simulink model "AuM_Ha5_A1"  (R2020a)
settings: Solver=VariableStepAuto  StartTime=0.0  StopTime=5  RelTol=1e-9
values from neighbouring files (symbols this model uses):
  J = 450e-6    (= 0.00045)    [AuM_HA05_A1_init.m]    (also in AuM_HA05_A2_init.m)
  L_S = 4e-3    (= 0.004)    [AuM_HA05_A1_init.m]    (also in AuM_HA05_A2_init.m)
  p = 5    [AuM_HA05_A1_init.m]    (also in AuM_HA05_A2_init.m)
  Psi_P = 4.5e-3    (= 0.0045)    [AuM_HA05_A1_init.m]    (also in AuM_HA05_A2_init.m)
  R_S = 0.58    [AuM_HA05_A1_init.m]    (also in AuM_HA05_A2_init.m)
  T_S = L_S/R_S    (= 0.00689655172414)    [AuM_HA05_A1_init.m]    (also in AuM_HA05_A2_init.m)
  U_d = 24    [AuM_HA05_A1_init.m]    (also in AuM_HA05_A2_init.m)
settings Model: Creator=Ravi Plenzdorf  LastModifiedBy=Ravi Plenzdorf

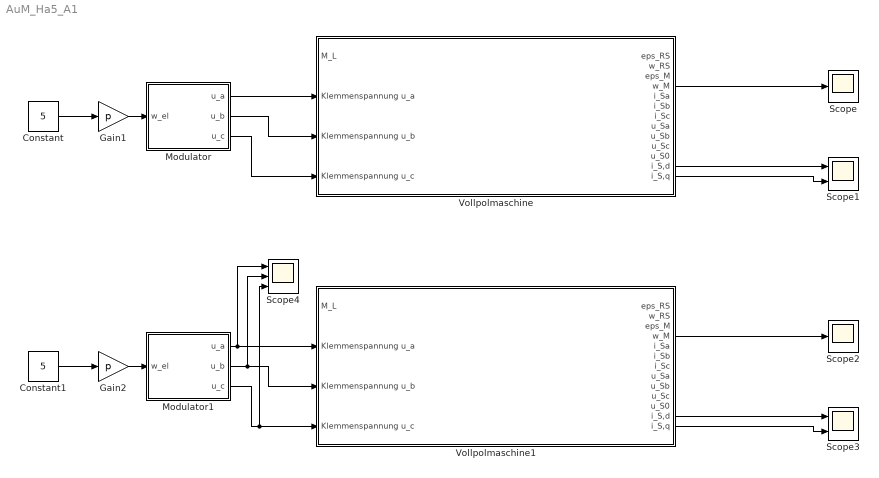
== system AuM_Ha5_A1 ==
  Constant : Constant  Value=5
  Constant1 : Constant  Value=5
  Gain1 : Gain  Gain=p
  Gain2 : Gain  Gain=p
  Modulator : Subsystem
  Modulator1 : Subsystem
  Scope : Scope
  Scope1 : Scope  NumInputPorts=2
  Scope2 : Scope
  Scope3 : Scope  NumInputPorts=2
  Scope4 : Scope  NumInputPorts=3
  Vollpolmaschine : Subsystem
      mask Display: image('Motor_Symbol.png'); % Use "Edit Image" on toolstrip to change.
  Vollpolmaschine1 : Subsystem
      mask Display: image('Motor_Symbol.png'); % Use "Edit Image" on toolstrip to change.
  wires:
  Vollpolmaschine/4(w_M) -> Scope/1
  Vollpolmaschine/12(i_S,d) -> Scope1/1
  Vollpolmaschine/13(i_S,q) -> Scope1/2
  Constant/1 -> Gain1/1
  Gain1/1 -> Modulator/1(w_el)
  Modulator/1(u_a) -> Vollpolmaschine/2(Klemmenspannung u_a)
  Modulator/2(u_b) -> Vollpolmaschine/3(Klemmenspannung u_b)
  Modulator/3(u_c) -> Vollpolmaschine/4(Klemmenspannung u_c)
  Modulator1/3(u_c) -> Scope4/3, Vollpolmaschine1/4(Klemmenspannung u_c)
  Modulator1/2(u_b) -> Scope4/2, Vollpolmaschine1/3(Klemmenspannung u_b)
  Modulator1/1(u_a) -> Vollpolmaschine1/2(Klemmenspannung u_a), Scope4/1
  Gain2/1 -> Modulator1/1(w_el)
  Constant1/1 -> Gain2/1
  Vollpolmaschine1/13(i_S,q) -> Scope3/2
  Vollpolmaschine1/12(i_S,d) -> Scope3/1
  Vollpolmaschine1/4(w_M) -> Scope2/1

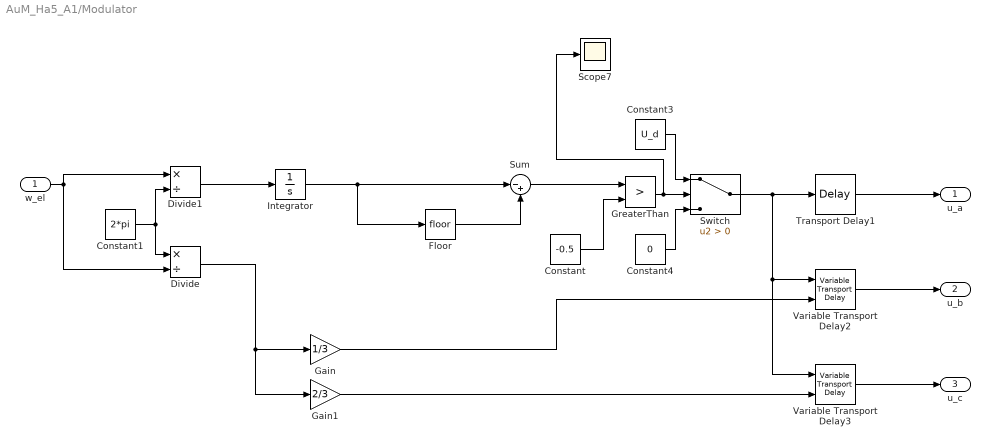
== system AuM_Ha5_A1/Modulator ==
  w_el : Inport
  Constant : Constant  Value=-0.5
  Constant1 : Constant  Value=2*pi
  Constant3 : Constant  Value=U_d
  Constant4 : Constant  Value=0
  Divide : Product  Inputs=*/
  Divide1 : Product  Inputs=*/
  Floor : Rounding
  Gain : Gain  Gain=1/3
  Gain1 : Gain  Gain=2/3
  GreaterThan : RelationalOperator  Operator=>  OutDataTypeStr=boolean  RndMeth=Simplest
  Integrator : Integrator
  Scope7 : Scope
  Sum : Sum  Inputs=|-+
  Switch : Switch  Criteria=u2 > Threshold
  Transport Delay1 : TransportDelay  DelayTime=0
  Variable Transport Delay2 : VariableTransportDelay  VariableDelayType=Variable transport delay  MaximumDelay=10
  Variable Transport Delay3 : VariableTransportDelay  VariableDelayType=Variable transport delay  MaximumDelay=10
  u_a : Outport
  u_b : Outport  Port=2
  u_c : Outport  Port=3
  wires:
  Constant4/1 -> Switch/3
  Constant3/1 -> Switch/1
  Sum/1 -> GreaterThan/1
  GreaterThan/1 -> Scope7/1, Switch/2
  Constant/1 -> GreaterThan/2
  Integrator/1 -> Floor/1, Sum/1
  Floor/1 -> Sum/2
  Switch/1 -> Variable Transport Delay3/1, Variable Transport Delay2/1, Transport Delay1/1
  w_el/1 -> Divide1/1, Divide/2
  Divide/1 -> Gain1/1, Gain/1
  Gain/1 -> Variable Transport Delay2/2
  Gain1/1 -> Variable Transport Delay3/2
  Constant1/1 -> Divide/1, Divide1/2
  Divide1/1 -> Integrator/1
  Transport Delay1/1 -> u_a/1
  Variable Transport Delay2/1 -> u_b/1
  Variable Transport Delay3/1 -> u_c/1

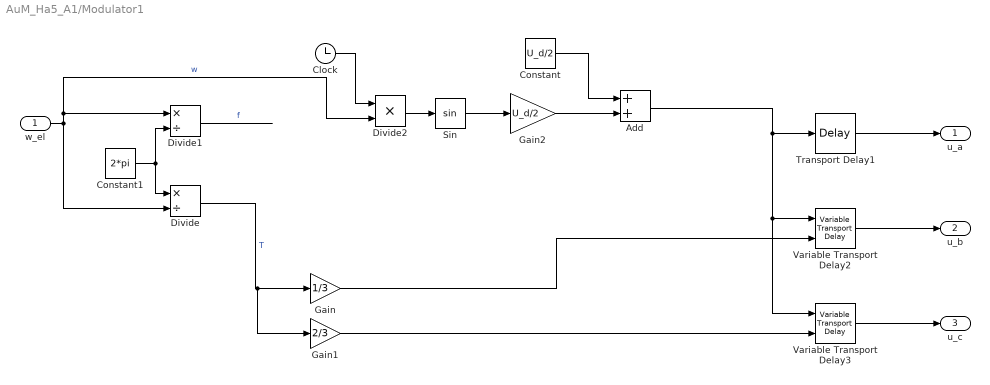
== system AuM_Ha5_A1/Modulator1 ==
  w_el : Inport
  Add : Sum
  Clock : Clock
  Constant : Constant  Value=U_d/2
  Constant1 : Constant  Value=2*pi
  Divide : Product  Inputs=*/
  Divide1 : Product  Inputs=*/
  Divide2 : Product  Inputs=**
  Gain : Gain  Gain=1/3
  Gain1 : Gain  Gain=2/3
  Gain2 : Gain  Gain=U_d/2
  Sin : Trigonometry
  Transport Delay1 : TransportDelay  DelayTime=0
  Variable Transport Delay2 : VariableTransportDelay  VariableDelayType=Variable transport delay  MaximumDelay=10
  Variable Transport Delay3 : VariableTransportDelay  VariableDelayType=Variable transport delay  MaximumDelay=10
  u_a : Outport
  u_b : Outport  Port=2
  u_c : Outport  Port=3
  wires:
  Variable Transport Delay3/1 -> u_c/1
  Variable Transport Delay2/1 -> u_b/1
  Transport Delay1/1 -> u_a/1
  Constant1/1 -> Divide1/2, Divide/1
  Gain/1 -> Variable Transport Delay2/2
  w_el/1 -> Divide2/2, Divide1/1, Divide/2  "w"
  Add/1 -> Transport Delay1/1, Variable Transport Delay2/1, Variable Transport Delay3/1
  Divide/1 -> Gain1/1, Gain/1  "T"
  Divide1/1 -> ?  "f"
  Gain1/1 -> Variable Transport Delay3/2
  Clock/1 -> Divide2/1
  Divide2/1 -> Sin/1
  Sin/1 -> Gain2/1
  Gain2/1 -> Add/2
  Constant/1 -> Add/1

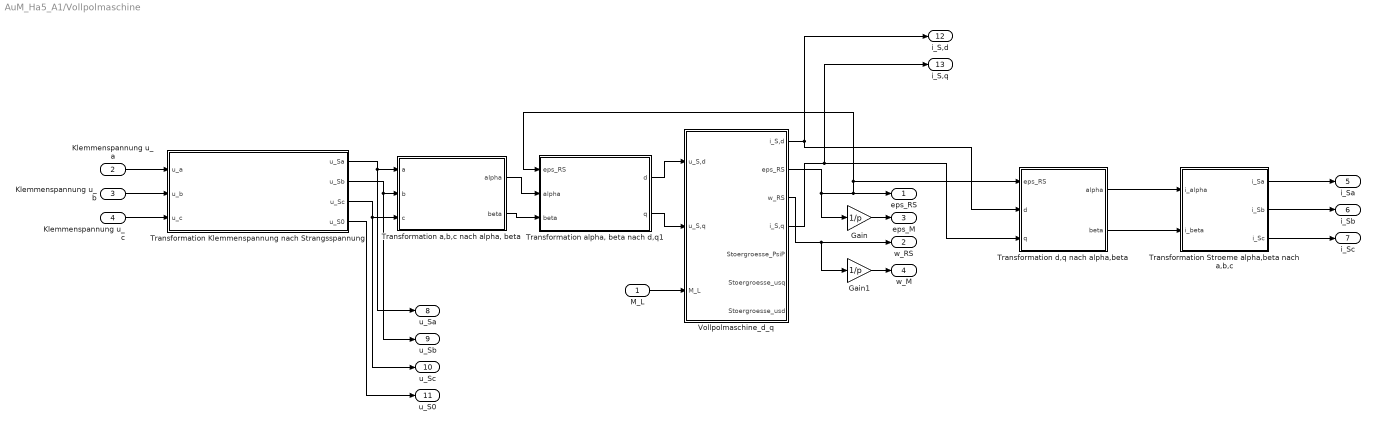
== system AuM_Ha5_A1/Vollpolmaschine ==
  M_L : Inport
  Klemmenspannung u_a : Inport  Port=2
  Klemmenspannung u_b : Inport  Port=3
  Klemmenspannung u_c : Inport  Port=4
  Gain : Gain  Gain=1/p
  Gain1 : Gain  Gain=1/p
  Transformation Klemmenspannung nach Strangsspannung : MATLAB Function  TreatAsAtomicUnit=on
  Transformation Stroeme alpha,beta nach a,b,c : MATLAB Function  TreatAsAtomicUnit=on
  "Transformation a,b,c nach alpha, beta" : MATLAB Function  TreatAsAtomicUnit=on
  "Transformation alpha, beta nach d,q1" : MATLAB Function  TreatAsAtomicUnit=on
  Transformation d,q nach alpha,beta : MATLAB Function  TreatAsAtomicUnit=on
  Vollpolmaschine_d_q : Subsystem
  eps_RS : Outport  VectorParamsAs1DForOutWhenUnconnected=off
  w_RS : Outport  Port=2  VectorParamsAs1DForOutWhenUnconnected=off
  eps_M : Outport  Port=3  VectorParamsAs1DForOutWhenUnconnected=off
  w_M : Outport  Port=4  VectorParamsAs1DForOutWhenUnconnected=off
  i_Sa : Outport  Port=5  VectorParamsAs1DForOutWhenUnconnected=off
  i_Sb : Outport  Port=6  VectorParamsAs1DForOutWhenUnconnected=off
  i_Sc : Outport  Port=7  VectorParamsAs1DForOutWhenUnconnected=off
  u_Sa : Outport  Port=8  VectorParamsAs1DForOutWhenUnconnected=off
  u_Sb : Outport  Port=9  VectorParamsAs1DForOutWhenUnconnected=off
  u_Sc : Outport  Port=10  VectorParamsAs1DForOutWhenUnconnected=off
  u_S0 : Outport  Port=11  VectorParamsAs1DForOutWhenUnconnected=off
  i_S,d : Outport  Port=12
  i_S,q : Outport  Port=13
  wires:
  Transformation Klemmenspannung nach Strangsspannung/4(u_S0) -> u_S0/1
  Transformation Stroeme alpha,beta nach a,b,c/3(i_Sc) -> i_Sc/1
  Transformation Stroeme alpha,beta nach a,b,c/2(i_Sb) -> i_Sb/1
  Transformation Stroeme alpha,beta nach a,b,c/1(i_Sa) -> i_Sa/1
  Transformation d,q nach alpha,beta/2(beta) -> Transformation Stroeme alpha,beta nach a,b,c/2(i_beta)
  Transformation d,q nach alpha,beta/1(alpha) -> Transformation Stroeme alpha,beta nach a,b,c/1(i_alpha)
  "Transformation alpha, beta nach d,q1"/1(d) -> Vollpolmaschine_d_q/1(u_S,d)
  Gain1/1 -> w_M/1
  Gain/1 -> eps_M/1
  Klemmenspannung u_c/1 -> Transformation Klemmenspannung nach Strangsspannung/3(u_c)
  Klemmenspannung u_b/1 -> Transformation Klemmenspannung nach Strangsspannung/2(u_b)
  Klemmenspannung u_a/1 -> Transformation Klemmenspannung nach Strangsspannung/1(u_a)
  "Transformation alpha, beta nach d,q1"/2(q) -> Vollpolmaschine_d_q/2(u_S,q)
  "Transformation a,b,c nach alpha, beta"/2(beta) -> "Transformation alpha, beta nach d,q1"/3(beta)
  "Transformation a,b,c nach alpha, beta"/1(alpha) -> "Transformation alpha, beta nach d,q1"/2(alpha)
  M_L/1 -> Vollpolmaschine_d_q/3(M_L)
  Transformation Klemmenspannung nach Strangsspannung/3(u_Sc) -> u_Sc/1, "Transformation a,b,c nach alpha, beta"/3(c)
  Vollpolmaschine_d_q/2(eps_RS) -> Gain/1, "Transformation alpha, beta nach d,q1"/1(eps_RS), Transformation d,q nach alpha,beta/1(eps_RS), eps_RS/1
  Transformation Klemmenspannung nach Strangsspannung/1(u_Sa) -> "Transformation a,b,c nach alpha, beta"/1(a), u_Sa/1
  Vollpolmaschine_d_q/3(w_RS) -> w_RS/1, Gain1/1
  Transformation Klemmenspannung nach Strangsspannung/2(u_Sb) -> "Transformation a,b,c nach alpha, beta"/2(b), u_Sb/1
  Vollpolmaschine_d_q/1(i_S,d) -> Transformation d,q nach alpha,beta/2(d), i_S,d/1
  Vollpolmaschine_d_q/4(i_S,q) -> Transformation d,q nach alpha,beta/3(q), i_S,q/1

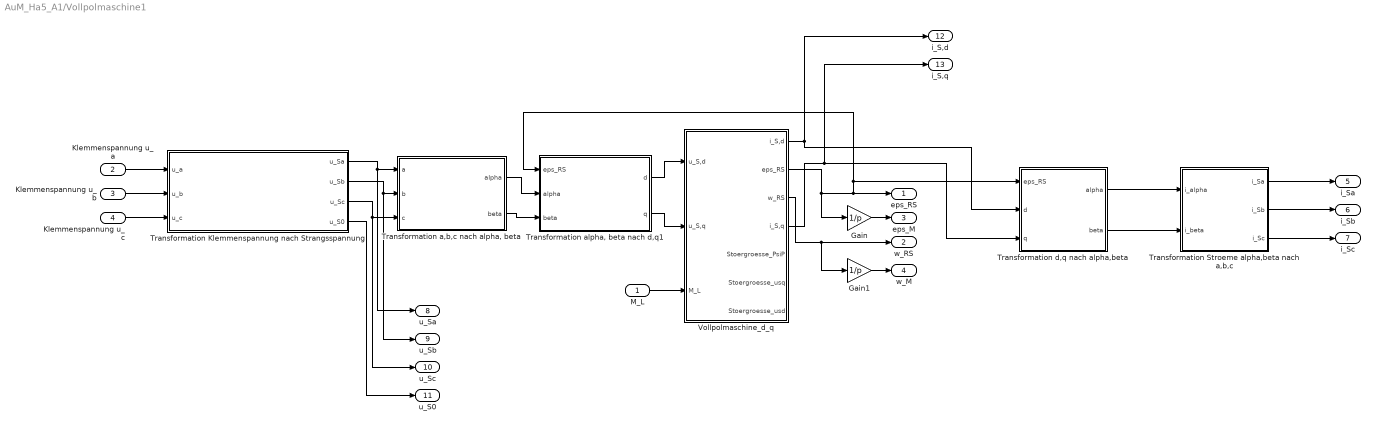
== system AuM_Ha5_A1/Vollpolmaschine1 ==
  M_L : Inport
  Klemmenspannung u_a : Inport  Port=2
  Klemmenspannung u_b : Inport  Port=3
  Klemmenspannung u_c : Inport  Port=4
  Gain : Gain  Gain=1/p
  Gain1 : Gain  Gain=1/p
  Transformation Klemmenspannung nach Strangsspannung : MATLAB Function  TreatAsAtomicUnit=on
  Transformation Stroeme alpha,beta nach a,b,c : MATLAB Function  TreatAsAtomicUnit=on
  "Transformation a,b,c nach alpha, beta" : MATLAB Function  TreatAsAtomicUnit=on
  "Transformation alpha, beta nach d,q1" : MATLAB Function  TreatAsAtomicUnit=on
  Transformation d,q nach alpha,beta : MATLAB Function  TreatAsAtomicUnit=on
  Vollpolmaschine_d_q : Subsystem
  eps_RS : Outport  VectorParamsAs1DForOutWhenUnconnected=off
  w_RS : Outport  Port=2  VectorParamsAs1DForOutWhenUnconnected=off
  eps_M : Outport  Port=3  VectorParamsAs1DForOutWhenUnconnected=off
  w_M : Outport  Port=4  VectorParamsAs1DForOutWhenUnconnected=off
  i_Sa : Outport  Port=5  VectorParamsAs1DForOutWhenUnconnected=off
  i_Sb : Outport  Port=6  VectorParamsAs1DForOutWhenUnconnected=off
  i_Sc : Outport  Port=7  VectorParamsAs1DForOutWhenUnconnected=off
  u_Sa : Outport  Port=8  VectorParamsAs1DForOutWhenUnconnected=off
  u_Sb : Outport  Port=9  VectorParamsAs1DForOutWhenUnconnected=off
  u_Sc : Outport  Port=10  VectorParamsAs1DForOutWhenUnconnected=off
  u_S0 : Outport  Port=11  VectorParamsAs1DForOutWhenUnconnected=off
  i_S,d : Outport  Port=12
  i_S,q : Outport  Port=13
  wires:
  Vollpolmaschine_d_q/4(i_S,q) -> i_S,q/1, Transformation d,q nach alpha,beta/3(q)
  Vollpolmaschine_d_q/1(i_S,d) -> i_S,d/1, Transformation d,q nach alpha,beta/2(d)
  Transformation Klemmenspannung nach Strangsspannung/2(u_Sb) -> u_Sb/1, "Transformation a,b,c nach alpha, beta"/2(b)
  Vollpolmaschine_d_q/3(w_RS) -> Gain1/1, w_RS/1
  Transformation Klemmenspannung nach Strangsspannung/1(u_Sa) -> u_Sa/1, "Transformation a,b,c nach alpha, beta"/1(a)
  Vollpolmaschine_d_q/2(eps_RS) -> eps_RS/1, Transformation d,q nach alpha,beta/1(eps_RS), "Transformation alpha, beta nach d,q1"/1(eps_RS), Gain/1
  Transformation Klemmenspannung nach Strangsspannung/3(u_Sc) -> "Transformation a,b,c nach alpha, beta"/3(c), u_Sc/1
  M_L/1 -> Vollpolmaschine_d_q/3(M_L)
  "Transformation a,b,c nach alpha, beta"/1(alpha) -> "Transformation alpha, beta nach d,q1"/2(alpha)
  "Transformation a,b,c nach alpha, beta"/2(beta) -> "Transformation alpha, beta nach d,q1"/3(beta)
  "Transformation alpha, beta nach d,q1"/2(q) -> Vollpolmaschine_d_q/2(u_S,q)
  Klemmenspannung u_a/1 -> Transformation Klemmenspannung nach Strangsspannung/1(u_a)
  Klemmenspannung u_b/1 -> Transformation Klemmenspannung nach Strangsspannung/2(u_b)
  Klemmenspannung u_c/1 -> Transformation Klemmenspannung nach Strangsspannung/3(u_c)
  Gain/1 -> eps_M/1
  Gain1/1 -> w_M/1
  "Transformation alpha, beta nach d,q1"/1(d) -> Vollpolmaschine_d_q/1(u_S,d)
  Transformation d,q nach alpha,beta/1(alpha) -> Transformation Stroeme alpha,beta nach a,b,c/1(i_alpha)
  Transformation d,q nach alpha,beta/2(beta) -> Transformation Stroeme alpha,beta nach a,b,c/2(i_beta)
  Transformation Stroeme alpha,beta nach a,b,c/1(i_Sa) -> i_Sa/1
  Transformation Stroeme alpha,beta nach a,b,c/2(i_Sb) -> i_Sb/1
  Transformation Stroeme alpha,beta nach a,b,c/3(i_Sc) -> i_Sc/1
  Transformation Klemmenspannung nach Strangsspannung/4(u_S0) -> u_S0/1

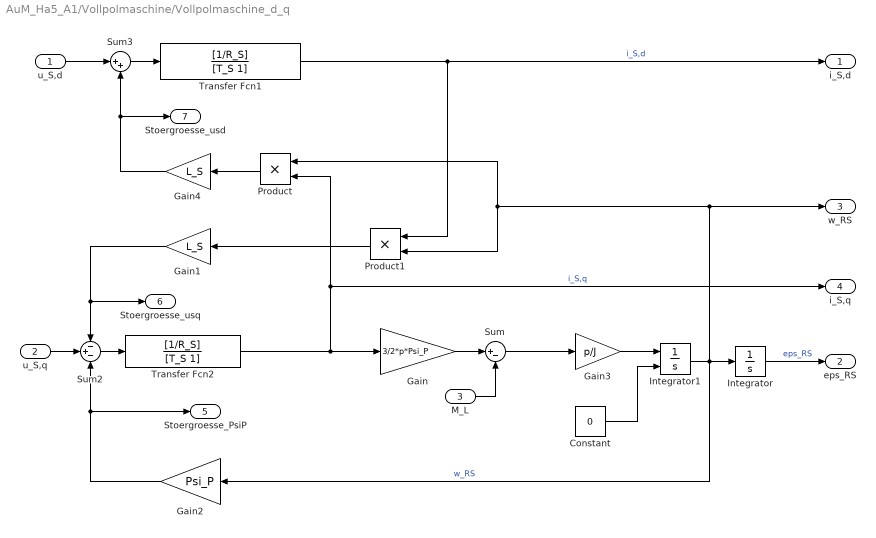
== system AuM_Ha5_A1/Vollpolmaschine/Vollpolmaschine_d_q ==
  u_S,d : Inport
  u_S,q : Inport  Port=2
  M_L : Inport  Port=3
  Constant : Constant  Value=0
  Gain : Gain  Gain=3/2*p*Psi_P
  Gain1 : Gain  Gain=L_S
  Gain2 : Gain  Gain=Psi_P
  Gain3 : Gain  Gain=p/J
  Gain4 : Gain  Gain=L_S
  Integrator : Integrator
  Integrator1 : Integrator  InitialConditionSource=external
  Product : Product
  Product1 : Product
  Sum : Sum  Inputs=|+-
  Sum2 : Sum  Inputs=-+-
  Sum3 : Sum  Inputs=|++
  Transfer Fcn1 : TransferFcn  Numerator=[1/R_S]  Denominator=[T_S 1]
  Transfer Fcn2 : TransferFcn  Numerator=[1/R_S]  Denominator=[T_S 1]
  i_S,d : Outport  VectorParamsAs1DForOutWhenUnconnected=off
  eps_RS : Outport  Port=2  VectorParamsAs1DForOutWhenUnconnected=off
  w_RS : Outport  Port=3  VectorParamsAs1DForOutWhenUnconnected=off
  i_S,q : Outport  Port=4  VectorParamsAs1DForOutWhenUnconnected=off
  Stoergroesse_PsiP : Outport  Port=5  VectorParamsAs1DForOutWhenUnconnected=off
  Stoergroesse_usq : Outport  Port=6  VectorParamsAs1DForOutWhenUnconnected=off
  Stoergroesse_usd : Outport  Port=7  VectorParamsAs1DForOutWhenUnconnected=off
  wires:
  Constant/1 -> Integrator1/2
  Transfer Fcn2/1 -> Product/2, i_S,q/1, Gain/1  "i_S,q"
  Gain4/1 -> Sum3/2, Stoergroesse_usd/1
  u_S,d/1 -> Sum3/1
  Gain1/1 -> Sum2/1, Stoergroesse_usq/1
  u_S,q/1 -> Sum2/2
  Product1/1 -> Gain1/1
  Transfer Fcn1/1 -> Product1/1, i_S,d/1  "i_S,d"
  Product/1 -> Gain4/1
  Sum3/1 -> Transfer Fcn1/1
  Gain2/1 -> Sum2/3, Stoergroesse_PsiP/1
  Gain3/1 -> Integrator1/1
  Gain/1 -> Sum/1
  M_L/1 -> Sum/2
  Sum/1 -> Gain3/1
  Integrator/1 -> eps_RS/1  "eps_RS"
  Integrator1/1 -> Gain2/1, Product1/2, Product/1, w_RS/1, Integrator/1  "w_RS"
  Sum2/1 -> Transfer Fcn2/1

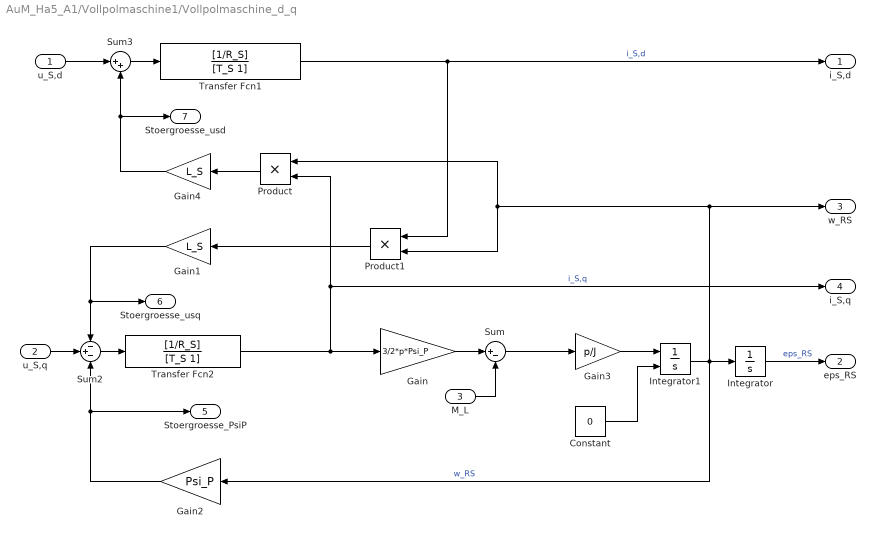
== system AuM_Ha5_A1/Vollpolmaschine1/Vollpolmaschine_d_q ==
  u_S,d : Inport
  u_S,q : Inport  Port=2
  M_L : Inport  Port=3
  Constant : Constant  Value=0
  Gain : Gain  Gain=3/2*p*Psi_P
  Gain1 : Gain  Gain=L_S
  Gain2 : Gain  Gain=Psi_P
  Gain3 : Gain  Gain=p/J
  Gain4 : Gain  Gain=L_S
  Integrator : Integrator
  Integrator1 : Integrator  InitialConditionSource=external
  Product : Product
  Product1 : Product
  Sum : Sum  Inputs=|+-
  Sum2 : Sum  Inputs=-+-
  Sum3 : Sum  Inputs=|++
  Transfer Fcn1 : TransferFcn  Numerator=[1/R_S]  Denominator=[T_S 1]
  Transfer Fcn2 : TransferFcn  Numerator=[1/R_S]  Denominator=[T_S 1]
  i_S,d : Outport  VectorParamsAs1DForOutWhenUnconnected=off
  eps_RS : Outport  Port=2  VectorParamsAs1DForOutWhenUnconnected=off
  w_RS : Outport  Port=3  VectorParamsAs1DForOutWhenUnconnected=off
  i_S,q : Outport  Port=4  VectorParamsAs1DForOutWhenUnconnected=off
  Stoergroesse_PsiP : Outport  Port=5  VectorParamsAs1DForOutWhenUnconnected=off
  Stoergroesse_usq : Outport  Port=6  VectorParamsAs1DForOutWhenUnconnected=off
  Stoergroesse_usd : Outport  Port=7  VectorParamsAs1DForOutWhenUnconnected=off
  wires:
  Sum2/1 -> Transfer Fcn2/1
  Integrator1/1 -> Integrator/1, w_RS/1, Product/1, Product1/2, Gain2/1  "w_RS"
  Integrator/1 -> eps_RS/1  "eps_RS"
  Sum/1 -> Gain3/1
  M_L/1 -> Sum/2
  Gain/1 -> Sum/1
  Gain3/1 -> Integrator1/1
  Gain2/1 -> Stoergroesse_PsiP/1, Sum2/3
  Sum3/1 -> Transfer Fcn1/1
  Product/1 -> Gain4/1
  Transfer Fcn1/1 -> i_S,d/1, Product1/1  "i_S,d"
  Product1/1 -> Gain1/1
  u_S,q/1 -> Sum2/2
  Gain1/1 -> Stoergroesse_usq/1, Sum2/1
  u_S,d/1 -> Sum3/1
  Gain4/1 -> Stoergroesse_usd/1, Sum3/2
  Transfer Fcn2/1 -> Gain/1, i_S,q/1, Product/2  "i_S,q"
  Constant/1 -> Integrator1/2

== matlab function AuM_Ha5_A1/Vollpolmaschine/Transformation d,q nach alpha,beta ==
  data: eps_RS input; alpha output; d input; q input; beta output
function [alpha,beta] = fcn(eps_RS,d,q)
%#codegen
In=[d;q];
Out=[cos(eps_RS) -sin(eps_RS);sin(eps_RS) cos(eps_RS)]*In;
alpha=Out(1);
beta=Out(2);

== matlab function AuM_Ha5_A1/Vollpolmaschine1/Transformation Klemmenspannung nach Strangsspannung ==
  data: u_a input; u_Sa output; u_b input; u_c input; u_Sb output; u_Sc output; u_S0 output
function [u_Sa,u_Sb,u_Sc,u_S0] = fcn(u_a,u_b,u_c)
%Konvertiert Klemmenspannungen in Strangspannungen
u_S0=u_a/3+u_b/3+u_c/3;
u_Sa=u_a-u_S0;
u_Sb=u_b-u_S0;
u_Sc=u_c-u_S0;
end

== matlab function AuM_Ha5_A1/Vollpolmaschine1/Transformation Stroeme alpha,beta nach a,b,c ==
  data: i_alpha input; i_Sa output; i_beta input; i_Sb output; i_Sc output
function [i_Sa,i_Sb,i_Sc] = fcn(i_alpha,i_beta)
%#codegen
In=[i_alpha;i_beta];
Mat=[1 0; -0.5 sqrt(3)/2];
Out=Mat*In;
i_Sa=Out(1);
i_Sb=Out(2);
i_Sc=-i_Sa-i_Sb;

== matlab function AuM_Ha5_A1/Vollpolmaschine1/Transformation a,b,c nach alpha, beta ==
  data: a input; alpha output; b input; c input; beta output
function [alpha,beta] = fcn(a,b,c)
In=[a;b;c];
Out=2/3*[1 -0.5 -0.5; 0 sqrt(3)/2 -sqrt(3)/2]*In;
alpha=Out(1);
beta=Out(2);

== matlab function AuM_Ha5_A1/Vollpolmaschine1/Transformation alpha, beta nach d,q1 ==
  data: eps_RS input; d output; alpha input; beta input; q output
function [d,q] = fcn(eps_RS,alpha,beta)
%#codegen
In=[alpha;beta];
Out=[cos(eps_RS) sin(eps_RS);-sin(eps_RS) cos(eps_RS)]*In;
d=Out(1);
q=Out(2);

== matlab function AuM_Ha5_A1/Vollpolmaschine1/Transformation d,q nach alpha,beta ==
  data: eps_RS input; alpha output; d input; q input; beta output
function [alpha,beta] = fcn(eps_RS,d,q)
%#codegen
In=[d;q];
Out=[cos(eps_RS) -sin(eps_RS);sin(eps_RS) cos(eps_RS)]*In;
alpha=Out(1);
beta=Out(2);

== matlab function AuM_Ha5_A1/Vollpolmaschine/Transformation Klemmenspannung nach Strangsspannung ==
  data: u_a input; u_Sa output; u_b input; u_c input; u_Sb output; u_Sc output; u_S0 output
function [u_Sa,u_Sb,u_Sc,u_S0] = fcn(u_a,u_b,u_c)
%Konvertiert Klemmenspannungen in Strangspannungen
u_S0=u_a/3+u_b/3+u_c/3;
u_Sa=u_a-u_S0;
u_Sb=u_b-u_S0;
u_Sc=u_c-u_S0;
end

== matlab function AuM_Ha5_A1/Vollpolmaschine/Transformation Stroeme alpha,beta nach a,b,c ==
  data: i_alpha input; i_Sa output; i_beta input; i_Sb output; i_Sc output
function [i_Sa,i_Sb,i_Sc] = fcn(i_alpha,i_beta)
%#codegen
In=[i_alpha;i_beta];
Mat=[1 0; -0.5 sqrt(3)/2];
Out=Mat*In;
i_Sa=Out(1);
i_Sb=Out(2);
i_Sc=-i_Sa-i_Sb;

== matlab function AuM_Ha5_A1/Vollpolmaschine/Transformation a,b,c nach alpha, beta ==
  data: a input; alpha output; b input; c input; beta output
function [alpha,beta] = fcn(a,b,c)
In=[a;b;c];
Out=2/3*[1 -0.5 -0.5; 0 sqrt(3)/2 -sqrt(3)/2]*In;
alpha=Out(1);
beta=Out(2);

== matlab function AuM_Ha5_A1/Vollpolmaschine/Transformation alpha, beta nach d,q1 ==
  data: eps_RS input; d output; alpha input; beta input; q output
function [d,q] = fcn(eps_RS,alpha,beta)
%#codegen
In=[alpha;beta];
Out=[cos(eps_RS) sin(eps_RS);-sin(eps_RS) cos(eps_RS)]*In;
d=Out(1);
q=Out(2);
